simulink model "IrSignalStateflow"  (R2022b)
settings: Solver=FixedStepAuto  StartTime=0.0  StopTime=inf  RelTol=1e-3  EnableMultiTasking=on
libraries: vexarmcortexlib x4
settings Model: ExtModeTrigDuration=25  Creator=Mihai Nicoara  LastModifiedBy=Mihai Nicoara
settings OptimizationCC: EnhancedBackFolding=on  PassReuseOutputArgsAs=Individual arguments  ZeroExternalMemoryAtStartup=off  ZeroInternalMemoryAtStartup=off  MaxStackSize=64  OptimizeBlockOrder=speed  DifferentSizesBufferReuse=on  OptimizationCustomize=off  EfficientTunableParamExpr=on
settings DebuggingCC: ParameterTunabilityLossMsg=error
settings HardwareCC: ProdBitPerPointer=32  ProdBitPerSizeT=32  ProdBitPerPtrDiffT=32  ProdLargestAtomicInteger=Long  ProdLargestAtomicFloat=Double  ProdWordSize=32  ProdHWDeviceType=ARM Compatible->ARM Cortex
settings SFSimCC: MATLABDynamicMemAlloc=off
settings RTWCC: Description=Embedded Coder  SystemTargetFile=ert.tlc  HardwareBoard=ARM Cortex-based VEX Microcontroller  TLCOptions="-aInlineSetEventsForThisBaseRateFcn=TLC_FALSE -aSuppressMultiTaskScheduler=TLC_FALSE  -aRateBasedStepFcn=0"  TemplateMakefile=ert_default_tmf  Toolchain=GNU Tools for VEX ARM Cortex
settings CodeAppCC: ForceParamTrailComments=on  IgnoreCustomStorageClasses=off  OperatorAnnotations=on  SimulinkDataObjDesc=on  SFDataObjDesc=on  InsertBlockDesc=on
settings ERTTargetCC: ExtModeTransport=1  ExtModeMexFile=ext_serial_win32_comm

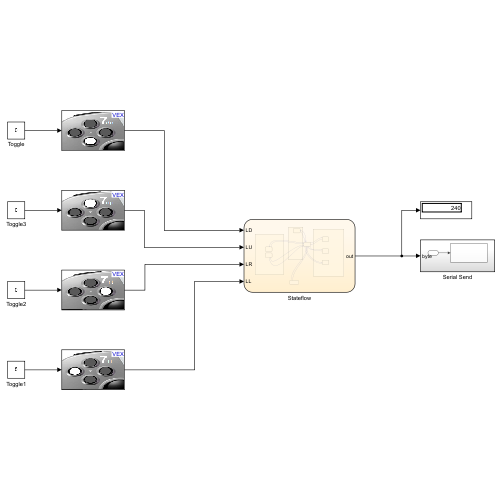
[thumbnail: Simulink's stored preview of the top-level diagram]
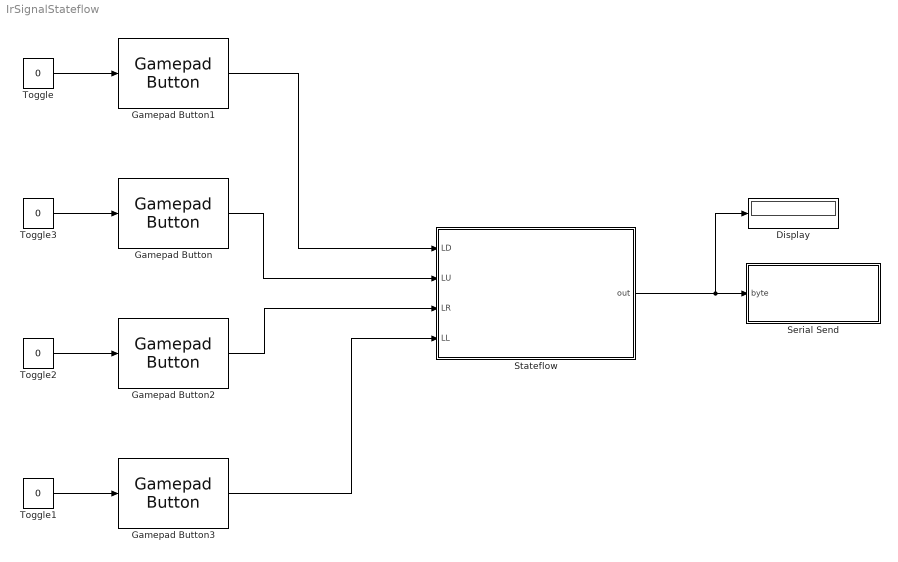
== system IrSignalStateflow ==
  Display : Display
  Gamepad Button : vexarmcortexlib/Gamepad/Gamepad Button  joystick=1  chan=7  button56=Up  button78=Up  SimulationIn=on  SampleTime=0.02
  Gamepad Button1 : vexarmcortexlib/Gamepad/Gamepad Button  joystick=1  chan=7  button56=Up  button78=Down  SimulationIn=on  SampleTime=0.02
  Gamepad Button2 : vexarmcortexlib/Gamepad/Gamepad Button  joystick=1  chan=7  button56=Up  button78=Right  SimulationIn=on  SampleTime=0.02
  Gamepad Button3 : vexarmcortexlib/Gamepad/Gamepad Button  joystick=1  chan=7  button56=Up  button78=Left  SimulationIn=on  SampleTime=0.02
  Serial Send : Subsystem
  Stateflow : Stateflow chart  TreatAsAtomicUnit=on
  Toggle{,1..3} (4 alike) : Constant  Value=0
      settings: OpenFcn=|
      | if strcmp('0',get_param(gcb, 'Value'))                        set_param(gcb, 'Value', '1');
      | else
      |             set_param(gcb, 'Value', '0');
      | end
  wires:
  Gamepad Button/1 -> Stateflow/2(LU)
  Stateflow/1(out) -> Display/1, Serial Send/1(byte)
  Gamepad Button2/1 -> Stateflow/3(LR)
  Gamepad Button3/1 -> Stateflow/4(LL)
  Gamepad Button1/1 -> Stateflow/1(LD)
  Toggle/1 -> Gamepad Button1/1
  Toggle3/1 -> Gamepad Button/1
  Toggle2/1 -> Gamepad Button2/1
  Toggle1/1 -> Gamepad Button3/1

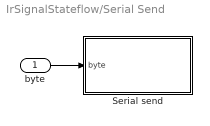
== system IrSignalStateflow/Serial Send ==
  byte : Inport  OutDataTypeStr=uint8  PortDimensions=[1 1]
  Serial send : MATLAB Function  TreatAsAtomicUnit=on
  wires:
  byte/1 -> Serial send/1(byte)

== stateflow chart IrSignalStateflow/Stateflow ==
  state Speed Adjustments [group]
    state speedHigh
      entry:
      out = 0xC3;
  state Squeaky Movements [group]
    state LiftMid
      entry:
      out = 0x5A;
    state driveMid
      entry:
      out = 0x33;
    state rotateMid
      entry:
      out = 0x66;
  state Rotational Adjustments [group]
    state rotLow
      entry:
      out = 0x69;
    state RotHigh
      entry:
      out = 0x0F;
  state Default_Flash
    entry:
    out = 0xF0;
  state MasterFeildReset
    entry:
    out = 0xAA;
  Default_Flash -> speedHigh [order 4] : [LL == 1 && LU == 1]
  speedHigh -> Default_Flash : [after(0.5,sec)]
  Default_Flash -> LiftMid [order 1] : [LL == 1]
  LiftMid -> Default_Flash : [after(0.5,sec)]
  (default) -> Default_Flash
  Default_Flash -> rotLow [order 5] : [LL == 1 && LR == 1]
  rotLow -> Default_Flash : [after(0.5,sec)]
  Default_Flash -> RotHigh [order 6] : [LU == 1 && LD == 1]
  RotHigh -> Default_Flash : [after(0.5,sec)]
  Default_Flash -> MasterFeildReset [order 7] : [LU == 1 && LD == 1 && LR == 1 && LL == 1]
  MasterFeildReset -> Default_Flash : [after(0.5,sec)]
  rotateMid -> Default_Flash : [after(0.5,sec)]
  Default_Flash -> rotateMid [order 3] : [LR == 1]
  driveMid -> Default_Flash : [after(0.5,sec)]
  Default_Flash -> driveMid [order 2] : [LD == 1]
  data: LD input; LU input; out output; LR input; LL input

== matlab function IrSignalStateflow/Serial Send/Serial send ==
  data: byte input
function fcn(byte)
% Serial send single byte
%#codegen

% Config
port = 'uart1';
baud = uint32(600);

persistent isFirstRun

if coder.target('Rtw')
    coder.cinclude('API.h');
    coder.cinclude('string.h');
    file = coder.opaque('FILE *', port,'HeaderFile','API.h');

    if isempty(isFirstRun)
        % first time setup
        isFirstRun = false;

        flags = coder.opaque('uint16', 'SERIAL_8N1');
        coder.ceval('usartInit', file, baud, flags);
    end

    coder.ceval('fputc', byte, file);

end

end
